simulink model "prob49c"  (R2018a)
settings: Solver=ode4  StartTime=0.0  StopTime=300.0  FixedStep=0.001  RelTol=1e-3
values from neighbouring files (symbols this model uses):
  A = [a11 a12 ... (first row only)    [p49cConsts.m]
  alfa = 3    [p49cConsts.m]
  B = [b1 ... (first row only)    [p49cConsts.m]
  lambda_0 = 3    [p49cConsts.m]
  lambda_1 = 0.1    [p49cConsts.m]
  P0 = [3 0 0 ... (first row only)    [p49cConsts.m]
  x0 = [0;0]    [p49cConsts.m]
settings Model: Creator=Kristian  LastModifiedBy=Kristian
settings CodeAppCC: StateflowObjectComments=on

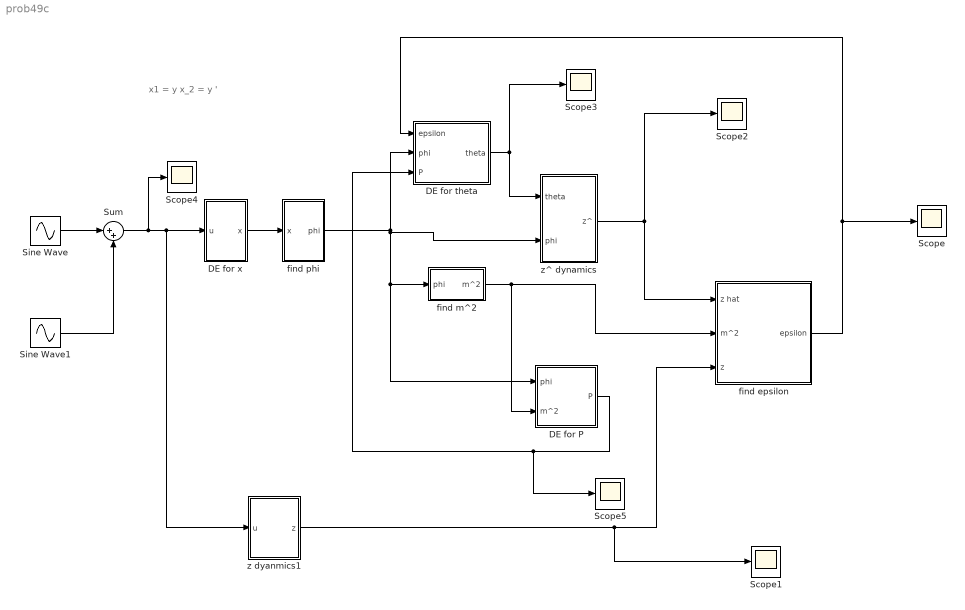
== system prob49c ==
  note: x1 = y
      | x_2 = y '
  DE for P : Subsystem
  DE for theta : Subsystem
  DE for x : Subsystem
  Scope{,1..5} (6 alike) : Scope
  Sine Wave : Sin  Amplitude=5  Phase=0.3  SampleTime=0
  Sine Wave1 : Sin  Amplitude=7  Frequency=2  SampleTime=0
  Sum : Sum  Inputs=|++
  find epsilon : Subsystem
  find m^2 : Subsystem
  find phi : Subsystem
  z dyanmics1 : Subsystem
  z^ dynamics : Subsystem
  wires:
  DE for x/1("x ") -> find phi/1(x)
  find phi/1("phi ") -> z^ dynamics/2(phi), DE for P/1("phi "), find m^2/1("phi "), DE for theta/2(phi)
  z^ dynamics/1("z^ ") -> Scope2/1, find epsilon/1(z hat)
  DE for theta/1("theta ") -> Scope3/1, z^ dynamics/1(theta)
  find epsilon/1("epsilon ") -> DE for theta/1("epsilon "), Scope/1
  z dyanmics1/1("z ") -> Scope1/1, find epsilon/3(z)
  find m^2/1("m^2 ") -> DE for P/2(m^2), find epsilon/2(m^2)
  DE for P/1("P ") -> Scope5/1, DE for theta/3(P)
  Sine Wave/1 -> Sum/1
  Sum/1 -> Scope4/1, z dyanmics1/1(u), DE for x/1(u)
  Sine Wave1/1 -> Sum/2

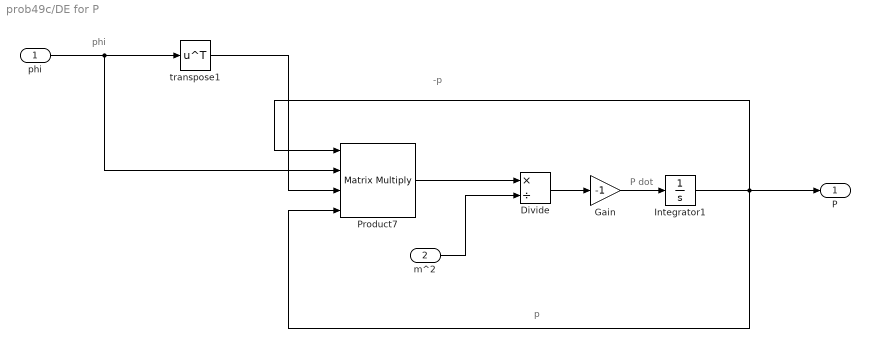
== system prob49c/DE for P ==
  note: P dot
  note: -p
  note: p
  note: phi
  "phi " : Inport
  m^2 : Inport  Port=2
  Divide : Product  Inputs=*/
  Gain : Gain  Gain=-1
  Integrator1 : Integrator  InitialCondition=P0
  Product7 : Product  Inputs=4  Multiplication=Matrix(*)
  transpose1 : Math  Operator=transpose  SaturateOnIntegerOverflow=on
  "P " : Outport
  wires:
  "phi "/1 -> Product7/2, transpose1/1
  transpose1/1 -> Product7/3
  Integrator1/1 -> Product7/4, Product7/1, "P "/1
  Product7/1 -> Divide/1
  m^2/1 -> Divide/2
  Divide/1 -> Gain/1
  Gain/1 -> Integrator1/1

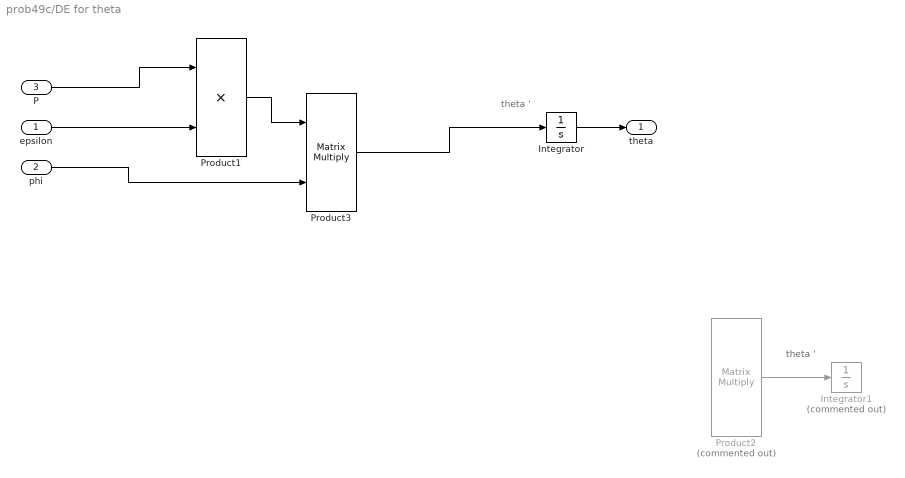
== system prob49c/DE for theta ==
  note: theta '
  note: theta '
  "epsilon " : Inport
  phi : Inport  Port=2
  P : Inport  Port=3
  Integrator : Integrator
  Integrator1 : Integrator  Commented=on
  Product1 : Product
  Product2 : Product  Commented=on  Inputs=3  Multiplication=Matrix(*)
  Product3 : Product  Multiplication=Matrix(*)
  "theta " : Outport
  wires:
  Integrator/1 -> "theta "/1
  P/1 -> Product1/1
  "epsilon "/1 -> Product1/2
  Product1/1 -> Product3/1
  phi/1 -> Product3/2
  Product3/1 -> Integrator/1
  Product2/1 -> Integrator1/1

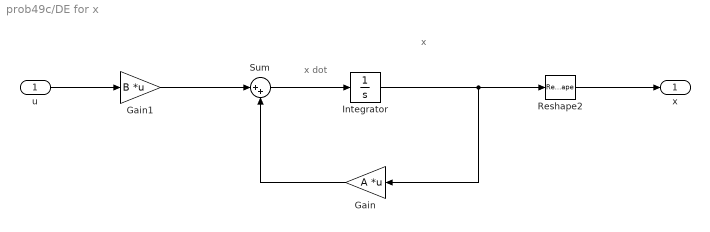
== system prob49c/DE for x ==
  note: x
  note: x dot
  u : Inport
  Gain : Gain  Gain=A  Multiplication=Matrix(K*u)
  Gain1 : Gain  Gain=B  Multiplication=Matrix(K*u)
  Integrator : Integrator  InitialCondition=x0
  Reshape2 : Reshape  OutputDimensionality=Column vector (2-D)
  Sum : Sum  Inputs=|++
  "x " : Outport
  wires:
  Gain/1 -> Sum/2
  u/1 -> Gain1/1
  Gain1/1 -> Sum/1
  Sum/1 -> Integrator/1
  Integrator/1 -> Reshape2/1, Gain/1
  Reshape2/1 -> "x "/1

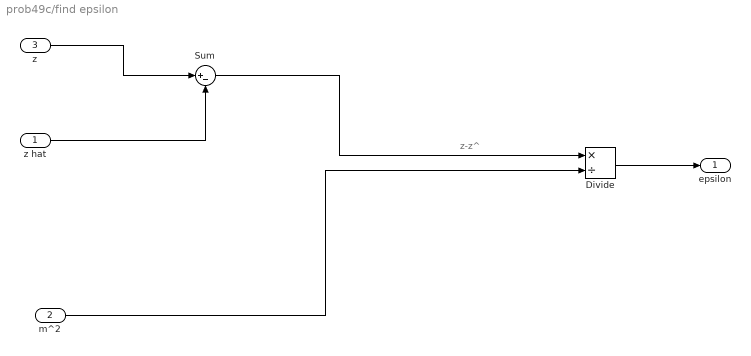
== system prob49c/find epsilon ==
  note: z-z^
  z hat : Inport
  m^2 : Inport  Port=2
  z : Inport  Port=3
  Divide : Product  Inputs=*/
  Sum : Sum  Inputs=|+-
  "epsilon " : Outport
  wires:
  z/1 -> Sum/1
  z hat/1 -> Sum/2
  m^2/1 -> Divide/2
  Sum/1 -> Divide/1
  Divide/1 -> "epsilon "/1

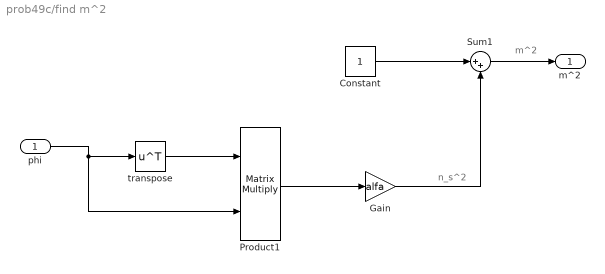
== system prob49c/find m^2 ==
  note: n_s^2
  note: m^2
  "phi " : Inport
  Constant : Constant
  Gain : Gain  Gain=alfa
  Product1 : Product  Multiplication=Matrix(*)
  Sum1 : Sum  Inputs=|++
  transpose : Math  Operator=transpose  SaturateOnIntegerOverflow=on
  "m^2 " : Outport
  wires:
  Constant/1 -> Sum1/1
  "phi "/1 -> Product1/2, transpose/1
  transpose/1 -> Product1/1
  Product1/1 -> Gain/1
  Gain/1 -> Sum1/2
  Sum1/1 -> "m^2 "/1

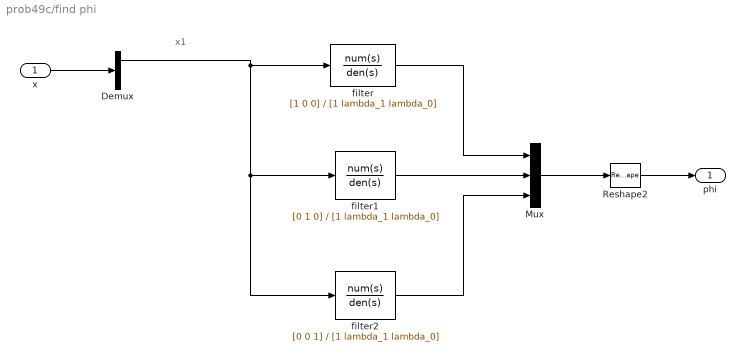
== system prob49c/find phi ==
  note: x1
  x : Inport
  Demux : Demux  Outputs=2
  Mux : Mux  Inputs=3
  Reshape2 : Reshape  OutputDimensionality=Column vector (2-D)
  filter : TransferFcn  Numerator=[1 0 0]  Denominator=[1 lambda_1 lambda_0]
  filter1 : TransferFcn  Numerator=[0 1 0]  Denominator=[1 lambda_1 lambda_0]
  filter2 : TransferFcn  Numerator=[0 0 1]  Denominator=[1 lambda_1 lambda_0]
  "phi " : Outport
  wires:
  x/1 -> Demux/1
  Demux/1 -> filter2/1, filter1/1, filter/1
  filter/1 -> Mux/1
  filter1/1 -> Mux/2
  filter2/1 -> Mux/3
  Mux/1 -> Reshape2/1
  Reshape2/1 -> "phi "/1

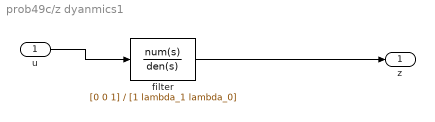
== system prob49c/z dyanmics1 ==
  u : Inport
  filter : TransferFcn  Numerator=[0 0 1]  Denominator=[1 lambda_1 lambda_0]
  "z " : Outport
  wires:
  u/1 -> filter/1
  filter/1 -> "z "/1

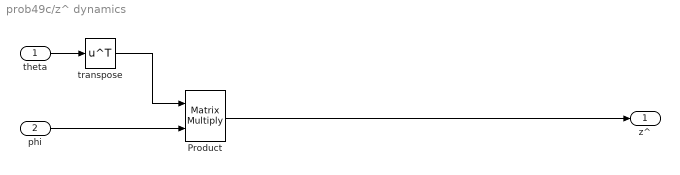
== system prob49c/z^ dynamics ==
  theta : Inport
  phi : Inport  Port=2
  Product : Product  Multiplication=Matrix(*)
  transpose : Math  Operator=transpose  SaturateOnIntegerOverflow=on
  "z^ " : Outport
  wires:
  Product/1 -> "z^ "/1
  theta/1 -> transpose/1
  transpose/1 -> Product/1
  phi/1 -> Product/2
